simulink model "Generic_13"  (R2022b)
settings: Solver=VariableStepAuto  StartTime=0.0  StopTime=10.0  RelTol=1e-3
values from neighbouring files (symbols this model uses):
  A = cell2mat(A_cell)    [MPCController1.m]    (also in MPC_Fmincon.m)
  B = cell2mat(B_cell)    [MPCController1.m]    (also in MPC_Fmincon.m)
  brake_select = ones(length(speed), length(steering_angle))    [TwoDLook_uptable.m]
  curvature = 0.000:0.001:1    [TwoDLook_uptable.m]
  m = 1600    [MPCController1.m]    (also in MPCController2.m; MPC_Fmincon.m)
  speed = 0:0.1:100    [TwoDLook_uptable.m]
undefined symbols (not defined in the file or in its folder): Amplifier, DiscIntNeverNeededParam, K_d_yawrate, K_dsteering, k_speed, k_stanley, kd, ki, kp, path_curvature
libraries: CarMaker4SL x121, simulink x12, cstblocks x7, autolibshared x1, mpcadaslib x1
(part 3 of 5)

== system Generic_13/CreateBus VhclCtrl/Stanley  steering & speed//Brake controller/Road sensor set & path planning/Road sensor set & path planning/Dijkestra path planning/Signal_smoothing ==
  Signal_In : Inport
  Smoothing1 : Subsystem
  Smoothing2 : Subsystem
  Smoothing4 : Subsystem
  smoothed_width : Outport
  wires:
  Smoothing4/1(Signal_Out) -> smoothed_width/1  "smoothed_width"
  Smoothing2/1(Signal_Out) -> Smoothing4/1(Signal_In)  "steering_signal"
  Smoothing1/1(Signal_Out) -> Smoothing2/1(Signal_In)  "steering_signal"
  Signal_In/1 -> Smoothing1/1(Signal_In)

== system Generic_13/CreateBus VhclCtrl/Stanley  steering & speed//Brake controller/Road sensor set & path planning/Road sensor set & path planning/Dijkestra path planning/Smoothing3 ==
  Signal_In : Inport
  Add : Sum  Inputs=++++
  Delay : Delay  InitialCondition=0.1
  Delay1 : Delay  DelayLength=4  InitialCondition=0.1
  Delay2 : Delay  DelayLength=5  InitialCondition=0.1
  Gain : Gain  Gain=0.35
  Gain1 : Gain  Gain=0.25
  Gain2 : Gain  Gain=0.25
  Gain3 : Gain  Gain=0.15
  Signal_Out : Outport  VectorParamsAs1DForOutWhenUnconnected=off
  wires:
  Gain1/1 -> Add/2
  Signal_In/1 -> Gain/1
  Delay/1 -> Gain1/1
  Gain/1 -> Add/1
  Delay1/1 -> Gain2/1
  Add/1 -> Delay2/1, Delay1/1, Delay/1, Signal_Out/1
  Gain2/1 -> Add/3
  Delay2/1 -> Gain3/1
  Gain3/1 -> Add/4

== system Generic_13/CreateBus VhclCtrl/Stanley  steering & speed//Brake controller/Road sensor set & path planning/Road sensor set & path planning/Path_curvature/ Path_expanding ==
  X-path : Inport
  Y_path : Inport  Port=2
  Delay10 : Delay  DelayLength=6
  Delay11 : Delay  DelayLength=8
  Delay37 : Delay
  Delay38 : Delay  DelayLength=4
  Delay4 : Delay
  Delay5 : Delay  DelayLength=6
  Delay6 : Delay  DelayLength=8
  Delay9 : Delay  DelayLength=4
  Mux1 : Mux  Inputs=5
  Mux2 : Mux  Inputs=5
  Reshape1 : Reshape  OutputDimensionality=Customize  OutputDimensions=[1,5]
  Reshape2 : Reshape  OutputDimensionality=Customize  OutputDimensions=[1,5]
  x_path : Outport
  y_path : Outport  Port=2
  wires:
  X-path/1 -> Mux2/1, Delay38/1, Delay37/1, Delay5/1, Delay6/1
  Y_path/1 -> Mux1/1, Delay4/1, Delay9/1, Delay10/1, Delay11/1
  Delay5/1 -> Mux2/4
  Delay37/1 -> Mux2/2
  Delay6/1 -> Mux2/5
  Delay38/1 -> Mux2/3
  Mux1/1 -> Reshape1/1
  Reshape1/1 -> y_path/1
  Delay4/1 -> Mux1/2
  Delay9/1 -> Mux1/3
  Delay10/1 -> Mux1/4
  Delay11/1 -> Mux1/5
  Reshape2/1 -> x_path/1
  Mux2/1 -> Reshape2/1

== system Generic_13/CreateBus VhclCtrl/Stanley  steering & speed//Brake controller/Road sensor set & path planning/Road sensor set & path planning/Spline_path_planning/Signal_smoothing ==
  Signal_In : Inport
  Smoothing1 : Subsystem
  Smoothing2 : Subsystem
  Smoothing4 : Subsystem
  smoothed_width : Outport
  wires:
  Signal_In/1 -> Smoothing1/1(Signal_In)
  Smoothing1/1(Signal_Out) -> Smoothing2/1(Signal_In)  "steering_signal"
  Smoothing2/1(Signal_Out) -> Smoothing4/1(Signal_In)  "steering_signal"
  Smoothing4/1(Signal_Out) -> smoothed_width/1  "smoothed_width"

== system Generic_13/CreateBus VhclCtrl/Stanley  steering & speed//Brake controller/Road sensor set & path planning/Road sensor set & path planning/Spline_path_planning/Smoothing3 ==
  Signal_In : Inport
  Add : Sum  Inputs=++++
  Delay : Delay  InitialCondition=0.1
  Delay1 : Delay  DelayLength=4  InitialCondition=0.1
  Delay2 : Delay  DelayLength=5  InitialCondition=0.1
  Gain : Gain  Gain=0.35
  Gain1 : Gain  Gain=0.25
  Gain2 : Gain  Gain=0.25
  Gain3 : Gain  Gain=0.15
  Signal_Out : Outport  VectorParamsAs1DForOutWhenUnconnected=off
  wires:
  Gain3/1 -> Add/4
  Delay2/1 -> Gain3/1
  Gain2/1 -> Add/3
  Add/1 -> Signal_Out/1, Delay/1, Delay1/1, Delay2/1
  Delay1/1 -> Gain2/1
  Gain/1 -> Add/1
  Delay/1 -> Gain1/1
  Signal_In/1 -> Gain/1
  Gain1/1 -> Add/2

== system Generic_13/CreateBus VhclCtrl/Stanley  steering & speed//Brake controller/Road sensor set & path planning/Road sensor set & path planning/path_planning/Signal_smoothing ==
  Signal_In : Inport
  Smoothing1 : Subsystem
  Smoothing2 : Subsystem
  Smoothing4 : Subsystem
  smoothed_width : Outport
  wires:
  Smoothing4/1(Signal_Out) -> smoothed_width/1  "smoothed_width"
  Smoothing2/1(Signal_Out) -> Smoothing4/1(Signal_In)  "steering_signal"
  Smoothing1/1(Signal_Out) -> Smoothing2/1(Signal_In)  "steering_signal"
  Signal_In/1 -> Smoothing1/1(Signal_In)

== system Generic_13/CreateBus VhclCtrl/Stanley  steering & speed//Brake controller/Road sensor set & path planning/Road sensor set & path planning/path_planning/Smoothing3 ==
  Signal_In : Inport
  Add : Sum  Inputs=++++
  Delay : Delay  InitialCondition=0.1
  Delay1 : Delay  DelayLength=4  InitialCondition=0.1
  Delay2 : Delay  DelayLength=5  InitialCondition=0.1
  Gain : Gain  Gain=0.35
  Gain1 : Gain  Gain=0.25
  Gain2 : Gain  Gain=0.25
  Gain3 : Gain  Gain=0.15
  Signal_Out : Outport  VectorParamsAs1DForOutWhenUnconnected=off
  wires:
  Gain1/1 -> Add/2
  Signal_In/1 -> Gain/1
  Delay/1 -> Gain1/1
  Gain/1 -> Add/1
  Delay1/1 -> Gain2/1
  Add/1 -> Delay2/1, Delay1/1, Delay/1, Signal_Out/1
  Gain2/1 -> Add/3
  Delay2/1 -> Gain3/1
  Gain3/1 -> Add/4

== system Generic_13/CreateBus VhclCtrl/Stanley  steering & speed//Brake controller/Stanley_controller_vfin/Stanley_controller_vfin/Stanley_standfort controller/Crosstrack_steering ==
  speed : Inport
  Path.DevDist : Inport  Port=2
  Atan : Trigonometry  Operator=atan
  Divide : Product  Inputs=*/
  Gain : Gain  Gain=-1
  Product : Product
  Sum1 : Sum  Inputs=|++
  k_speed : Constant  Value=k_speed
  k_stanley : Constant  Value=k_stanley
  Cross_track_steering : Outport
  wires:
  Atan/1 -> Cross_track_steering/1
  Divide/1 -> Atan/1
  k_speed/1 -> Sum1/1
  speed/1 -> Sum1/2
  k_stanley/1 -> Product/2
  Sum1/1 -> Divide/2
  Product/1 -> Gain/1
  Gain/1 -> Divide/1
  Path.DevDist/1 -> Product/1

== system Generic_13/CreateBus VhclCtrl/Stanley  steering & speed//Brake controller/Stanley_controller_vfin/Stanley_controller_vfin/Stanley_standfort controller/Deviation_angle_calc ==
  Velocity : Inport
  Curvature : Inport  Port=2
  Car.YawRate : Inport  Port=3
  Amplifyer : Gain  Gain=Amplifier
  Amplifyer1 : Gain  Gain=10
  Amplifyer2 : Gain  Gain=16.56
  Constant : Constant  Value=2
  Discrete-Time Integrator : DiscreteIntegrator  SampleTime=-1  ICPrevOutput=DiscIntNeverNeededParam  ICPrevScaledInput=DiscIntNeverNeededParam
  Integrator : DiscreteIntegrator  SampleTime=-1  ICPrevOutput=DiscIntNeverNeededParam  ICPrevScaledInput=DiscIntNeverNeededParam
  Multiport Switch : MultiPortSwitch  Inputs=2  SaturateOnIntegerOverflow=off  InputSameDT=off
  Product : Product
  Read CM Dict : CarMaker4SL/Read CM Dict  xname=Sensor.Road.VehSensor_0.Path.DevAng  xsync=off  xstime=Continuous
  Scope : Scope  NumInputPorts=2
  Sum3 : Sum  Inputs=|+-
  Switch : Switch  Criteria=u2 > Threshold  SaturateOnIntegerOverflow=off  InputSameDT=off
  Dev_angle : Outport
  wires:
  Amplifyer1/1 -> Switch/3  "Dev_angle"
  Curvature/1 -> Product/1
  Car.YawRate/1 -> Discrete-Time Integrator/1
  Velocity/1 -> Product/2
  Product/1 -> Integrator/1
  Integrator/1 -> Sum3/1  "Dev_angle"
  Discrete-Time Integrator/1 -> Sum3/2
  Amplifyer2/1 -> Switch/1  "Dev_angle"
  Sum3/1 -> Amplifyer1/1, Switch/2, Amplifyer2/1  "heading_error"
  Switch/1 -> Scope/1, Multiport Switch/2  "Dev_angle"
  Amplifyer/1 -> Scope/2, Multiport Switch/3  "Dev_angle"
  Read CM Dict/1 -> Amplifyer/1
  Constant/1 -> Multiport Switch/1
  Multiport Switch/1 -> Dev_angle/1  "Dev_angle"

== system Generic_13/CreateBus VhclCtrl/Stanley  steering & speed//Brake controller/Stanley_controller_vfin/Stanley_controller_vfin/Stanley_standfort controller/Steady_state_yaw ==
  V : Inport
  Curvature : Inport  Port=2
  Car_Yaw_rate : Inport  Port=3
  Discrete-Time Integrator : DiscreteIntegrator  SampleTime=-1  ICPrevOutput=DiscIntNeverNeededParam  ICPrevScaledInput=DiscIntNeverNeededParam
  Steady_state_yaw : Subsystem
  Sum : Sum  Inputs=|-+
  Steady_state_yaw1 : Outport
  wires:
  V/1 -> Steady_state_yaw/1(V)
  Sum/1 -> Steady_state_yaw1/1  "Steady_state_yaw"
  Steady_state_yaw/1(Steady_state_yaw) -> Sum/1  "Steady_state_yaw"
  Discrete-Time Integrator/1 -> Sum/2
  Car_Yaw_rate/1 -> Discrete-Time Integrator/1
  Curvature/1 -> Steady_state_yaw/2(Curvature)

== system Generic_13/CreateBus VhclCtrl/Stanley  steering & speed//Brake controller/Stanley_controller_vfin/Stanley_controller_vfin/Stanley_standfort controller/Steering_correction_facotr ==
  Steering_i+1 : Inport
  Steering_i : Inport  Port=2
  K_dsteering : Constant  Value=K_dsteering
  Memory : Memory  LinearizeAsDelay=on
  Product2 : Product
  Sum2 : Sum  Inputs=|+-
  Factor_of_correction : Outport
  wires:
  K_dsteering/1 -> Product2/1
  Memory/1 -> Sum2/1
  Sum2/1 -> Product2/2
  Steering_i+1/1 -> Sum2/2
  Steering_i/1 -> Memory/1
  Product2/1 -> Factor_of_correction/1

== system Generic_13/CreateBus VhclCtrl/Stanley  steering & speed//Brake controller/Stanley_controller_vfin/Stanley_controller_vfin/Stanley_standfort controller/Yaw_rate_diff ==
  Velocity : Inport
  Curvature : Inport  Port=2
  Car_yaw_rate : Inport  Port=3
  K_d_yawrate : Constant  Value=K_d_yawrate
  Product : Product
  Product1 : Product
  Sum1 : Sum  Inputs=|+-
  Yaw_rate_factor : Outport
  wires:
  K_d_yawrate/1 -> Product1/1
  Car_yaw_rate/1 -> Sum1/2
  Velocity/1 -> Product/1
  Curvature/1 -> Product/2
  Sum1/1 -> Product1/2
  Product/1 -> Sum1/1
  Product1/1 -> Yaw_rate_factor/1

== system Generic_13/CreateBus VhclCtrl/Stanley  steering & speed//Brake controller/Road sensor set & path planning/Road sensor set & path planning/A* star path planning/Signal_smoothing/Smoothing1 ==
  Signal_In : Inport
  Add : Sum  Inputs=++++
  Delay : Delay  InitialCondition=0.1
  Delay1 : Delay  DelayLength=4  InitialCondition=0.1
  Delay2 : Delay  DelayLength=5  InitialCondition=0.1
  Gain : Gain  Gain=0.35
  Gain1 : Gain  Gain=0.25
  Gain2 : Gain  Gain=0.25
  Gain3 : Gain  Gain=0.15
  Signal_Out : Outport  VectorParamsAs1DForOutWhenUnconnected=off
  wires:
  Gain1/1 -> Add/2
  Signal_In/1 -> Gain/1
  Delay/1 -> Gain1/1
  Gain/1 -> Add/1
  Delay1/1 -> Gain2/1
  Add/1 -> Delay2/1, Delay1/1, Delay/1, Signal_Out/1
  Gain2/1 -> Add/3
  Delay2/1 -> Gain3/1
  Gain3/1 -> Add/4

== system Generic_13/CreateBus VhclCtrl/Stanley  steering & speed//Brake controller/Road sensor set & path planning/Road sensor set & path planning/A* star path planning/Signal_smoothing/Smoothing2 ==
  Signal_In : Inport
  Add : Sum  Inputs=++++
  Delay : Delay  InitialCondition=0.1
  Delay1 : Delay  DelayLength=4  InitialCondition=0.1
  Delay2 : Delay  DelayLength=5  InitialCondition=0.1
  Gain : Gain  Gain=0.35
  Gain1 : Gain  Gain=0.25
  Gain2 : Gain  Gain=0.25
  Gain3 : Gain  Gain=0.15
  Signal_Out : Outport  VectorParamsAs1DForOutWhenUnconnected=off
  wires:
  Gain3/1 -> Add/4
  Delay2/1 -> Gain3/1
  Gain2/1 -> Add/3
  Add/1 -> Signal_Out/1, Delay/1, Delay1/1, Delay2/1
  Delay1/1 -> Gain2/1
  Gain/1 -> Add/1
  Delay/1 -> Gain1/1
  Signal_In/1 -> Gain/1
  Gain1/1 -> Add/2

== system Generic_13/CreateBus VhclCtrl/Stanley  steering & speed//Brake controller/Road sensor set & path planning/Road sensor set & path planning/A* star path planning/Signal_smoothing/Smoothing4 ==
  Signal_In : Inport
  Add : Sum  Inputs=++++
  Delay : Delay  InitialCondition=0.1
  Delay1 : Delay  DelayLength=4  InitialCondition=0.1
  Delay2 : Delay  DelayLength=5  InitialCondition=0.1
  Gain : Gain  Gain=0.35
  Gain1 : Gain  Gain=0.25
  Gain2 : Gain  Gain=0.25
  Gain3 : Gain  Gain=0.15
  Signal_Out : Outport  VectorParamsAs1DForOutWhenUnconnected=off
  wires:
  Gain1/1 -> Add/2
  Signal_In/1 -> Gain/1
  Delay/1 -> Gain1/1
  Gain/1 -> Add/1
  Delay1/1 -> Gain2/1
  Add/1 -> Delay2/1, Delay1/1, Delay/1, Signal_Out/1
  Gain2/1 -> Add/3
  Delay2/1 -> Gain3/1
  Gain3/1 -> Add/4

== system Generic_13/CreateBus VhclCtrl/Stanley  steering & speed//Brake controller/Road sensor set & path planning/Road sensor set & path planning/Be'zeir path planning/Signal_smoothing/Smoothing1 ==
  Signal_In : Inport
  Add : Sum  Inputs=++++
  Delay : Delay  InitialCondition=0.1
  Delay1 : Delay  DelayLength=4  InitialCondition=0.1
  Delay2 : Delay  DelayLength=5  InitialCondition=0.1
  Gain : Gain  Gain=0.35
  Gain1 : Gain  Gain=0.25
  Gain2 : Gain  Gain=0.25
  Gain3 : Gain  Gain=0.15
  Signal_Out : Outport  VectorParamsAs1DForOutWhenUnconnected=off
  wires:
  Gain3/1 -> Add/4
  Delay2/1 -> Gain3/1
  Gain2/1 -> Add/3
  Add/1 -> Signal_Out/1, Delay/1, Delay1/1, Delay2/1
  Delay1/1 -> Gain2/1
  Gain/1 -> Add/1
  Delay/1 -> Gain1/1
  Signal_In/1 -> Gain/1
  Gain1/1 -> Add/2

== system Generic_13/CreateBus VhclCtrl/Stanley  steering & speed//Brake controller/Road sensor set & path planning/Road sensor set & path planning/Be'zeir path planning/Signal_smoothing/Smoothing2 ==
  Signal_In : Inport
  Add : Sum  Inputs=++++
  Delay : Delay  InitialCondition=0.1
  Delay1 : Delay  DelayLength=4  InitialCondition=0.1
  Delay2 : Delay  DelayLength=5  InitialCondition=0.1
  Gain : Gain  Gain=0.35
  Gain1 : Gain  Gain=0.25
  Gain2 : Gain  Gain=0.25
  Gain3 : Gain  Gain=0.15
  Signal_Out : Outport  VectorParamsAs1DForOutWhenUnconnected=off
  wires:
  Gain1/1 -> Add/2
  Signal_In/1 -> Gain/1
  Delay/1 -> Gain1/1
  Gain/1 -> Add/1
  Delay1/1 -> Gain2/1
  Add/1 -> Delay2/1, Delay1/1, Delay/1, Signal_Out/1
  Gain2/1 -> Add/3
  Delay2/1 -> Gain3/1
  Gain3/1 -> Add/4

== system Generic_13/CreateBus VhclCtrl/Stanley  steering & speed//Brake controller/Road sensor set & path planning/Road sensor set & path planning/Be'zeir path planning/Signal_smoothing/Smoothing4 ==
  Signal_In : Inport
  Add : Sum  Inputs=++++
  Delay : Delay  InitialCondition=0.1
  Delay1 : Delay  DelayLength=4  InitialCondition=0.1
  Delay2 : Delay  DelayLength=5  InitialCondition=0.1
  Gain : Gain  Gain=0.35
  Gain1 : Gain  Gain=0.25
  Gain2 : Gain  Gain=0.25
  Gain3 : Gain  Gain=0.15
  Signal_Out : Outport  VectorParamsAs1DForOutWhenUnconnected=off
  wires:
  Gain3/1 -> Add/4
  Delay2/1 -> Gain3/1
  Gain2/1 -> Add/3
  Add/1 -> Signal_Out/1, Delay/1, Delay1/1, Delay2/1
  Delay1/1 -> Gain2/1
  Gain/1 -> Add/1
  Delay/1 -> Gain1/1
  Signal_In/1 -> Gain/1
  Gain1/1 -> Add/2

== system Generic_13/CreateBus VhclCtrl/Stanley  steering & speed//Brake controller/Road sensor set & path planning/Road sensor set & path planning/Dijkestra path planning/Signal_smoothing/Smoothing1 ==
  Signal_In : Inport
  Add : Sum  Inputs=++++
  Delay : Delay  InitialCondition=0.1
  Delay1 : Delay  DelayLength=4  InitialCondition=0.1
  Delay2 : Delay  DelayLength=5  InitialCondition=0.1
  Gain : Gain  Gain=0.35
  Gain1 : Gain  Gain=0.25
  Gain2 : Gain  Gain=0.25
  Gain3 : Gain  Gain=0.15
  Signal_Out : Outport  VectorParamsAs1DForOutWhenUnconnected=off
  wires:
  Gain3/1 -> Add/4
  Delay2/1 -> Gain3/1
  Gain2/1 -> Add/3
  Add/1 -> Signal_Out/1, Delay/1, Delay1/1, Delay2/1
  Delay1/1 -> Gain2/1
  Gain/1 -> Add/1
  Delay/1 -> Gain1/1
  Signal_In/1 -> Gain/1
  Gain1/1 -> Add/2

== system Generic_13/CreateBus VhclCtrl/Stanley  steering & speed//Brake controller/Road sensor set & path planning/Road sensor set & path planning/Dijkestra path planning/Signal_smoothing/Smoothing2 ==
  Signal_In : Inport
  Add : Sum  Inputs=++++
  Delay : Delay  InitialCondition=0.1
  Delay1 : Delay  DelayLength=4  InitialCondition=0.1
  Delay2 : Delay  DelayLength=5  InitialCondition=0.1
  Gain : Gain  Gain=0.35
  Gain1 : Gain  Gain=0.25
  Gain2 : Gain  Gain=0.25
  Gain3 : Gain  Gain=0.15
  Signal_Out : Outport  VectorParamsAs1DForOutWhenUnconnected=off
  wires:
  Gain1/1 -> Add/2
  Signal_In/1 -> Gain/1
  Delay/1 -> Gain1/1
  Gain/1 -> Add/1
  Delay1/1 -> Gain2/1
  Add/1 -> Delay2/1, Delay1/1, Delay/1, Signal_Out/1
  Gain2/1 -> Add/3
  Delay2/1 -> Gain3/1
  Gain3/1 -> Add/4

== system Generic_13/CreateBus VhclCtrl/Stanley  steering & speed//Brake controller/Road sensor set & path planning/Road sensor set & path planning/Dijkestra path planning/Signal_smoothing/Smoothing4 ==
  Signal_In : Inport
  Add : Sum  Inputs=++++
  Delay : Delay  InitialCondition=0.1
  Delay1 : Delay  DelayLength=4  InitialCondition=0.1
  Delay2 : Delay  DelayLength=5  InitialCondition=0.1
  Gain : Gain  Gain=0.35
  Gain1 : Gain  Gain=0.25
  Gain2 : Gain  Gain=0.25
  Gain3 : Gain  Gain=0.15
  Signal_Out : Outport  VectorParamsAs1DForOutWhenUnconnected=off
  wires:
  Gain3/1 -> Add/4
  Delay2/1 -> Gain3/1
  Gain2/1 -> Add/3
  Add/1 -> Signal_Out/1, Delay/1, Delay1/1, Delay2/1
  Delay1/1 -> Gain2/1
  Gain/1 -> Add/1
  Delay/1 -> Gain1/1
  Signal_In/1 -> Gain/1
  Gain1/1 -> Add/2

== system Generic_13/CreateBus VhclCtrl/Stanley  steering & speed//Brake controller/Road sensor set & path planning/Road sensor set & path planning/Spline_path_planning/Signal_smoothing/Smoothing1 ==
  Signal_In : Inport
  Add : Sum  Inputs=++++
  Delay : Delay  InitialCondition=0.1
  Delay1 : Delay  DelayLength=4  InitialCondition=0.1
  Delay2 : Delay  DelayLength=5  InitialCondition=0.1
  Gain : Gain  Gain=0.35
  Gain1 : Gain  Gain=0.25
  Gain2 : Gain  Gain=0.25
  Gain3 : Gain  Gain=0.15
  Signal_Out : Outport  VectorParamsAs1DForOutWhenUnconnected=off
  wires:
  Gain1/1 -> Add/2
  Signal_In/1 -> Gain/1
  Delay/1 -> Gain1/1
  Gain/1 -> Add/1
  Delay1/1 -> Gain2/1
  Add/1 -> Delay2/1, Delay1/1, Delay/1, Signal_Out/1
  Gain2/1 -> Add/3
  Delay2/1 -> Gain3/1
  Gain3/1 -> Add/4

== system Generic_13/CreateBus VhclCtrl/Stanley  steering & speed//Brake controller/Road sensor set & path planning/Road sensor set & path planning/Spline_path_planning/Signal_smoothing/Smoothing2 ==
  Signal_In : Inport
  Add : Sum  Inputs=++++
  Delay : Delay  InitialCondition=0.1
  Delay1 : Delay  DelayLength=4  InitialCondition=0.1
  Delay2 : Delay  DelayLength=5  InitialCondition=0.1
  Gain : Gain  Gain=0.35
  Gain1 : Gain  Gain=0.25
  Gain2 : Gain  Gain=0.25
  Gain3 : Gain  Gain=0.15
  Signal_Out : Outport  VectorParamsAs1DForOutWhenUnconnected=off
  wires:
  Gain3/1 -> Add/4
  Delay2/1 -> Gain3/1
  Gain2/1 -> Add/3
  Add/1 -> Signal_Out/1, Delay/1, Delay1/1, Delay2/1
  Delay1/1 -> Gain2/1
  Gain/1 -> Add/1
  Delay/1 -> Gain1/1
  Signal_In/1 -> Gain/1
  Gain1/1 -> Add/2

== system Generic_13/CreateBus VhclCtrl/Stanley  steering & speed//Brake controller/Road sensor set & path planning/Road sensor set & path planning/Spline_path_planning/Signal_smoothing/Smoothing4 ==
  Signal_In : Inport
  Add : Sum  Inputs=++++
  Delay : Delay  InitialCondition=0.1
  Delay1 : Delay  DelayLength=4  InitialCondition=0.1
  Delay2 : Delay  DelayLength=5  InitialCondition=0.1
  Gain : Gain  Gain=0.35
  Gain1 : Gain  Gain=0.25
  Gain2 : Gain  Gain=0.25
  Gain3 : Gain  Gain=0.15
  Signal_Out : Outport  VectorParamsAs1DForOutWhenUnconnected=off
  wires:
  Gain1/1 -> Add/2
  Signal_In/1 -> Gain/1
  Delay/1 -> Gain1/1
  Gain/1 -> Add/1
  Delay1/1 -> Gain2/1
  Add/1 -> Delay2/1, Delay1/1, Delay/1, Signal_Out/1
  Gain2/1 -> Add/3
  Delay2/1 -> Gain3/1
  Gain3/1 -> Add/4

== system Generic_13/CreateBus VhclCtrl/Stanley  steering & speed//Brake controller/Road sensor set & path planning/Road sensor set & path planning/path_planning/Signal_smoothing/Smoothing1 ==
  Signal_In : Inport
  Add : Sum  Inputs=++++
  Delay : Delay  InitialCondition=0.1
  Delay1 : Delay  DelayLength=4  InitialCondition=0.1
  Delay2 : Delay  DelayLength=5  InitialCondition=0.1
  Gain : Gain  Gain=0.35
  Gain1 : Gain  Gain=0.25
  Gain2 : Gain  Gain=0.25
  Gain3 : Gain  Gain=0.15
  Signal_Out : Outport  VectorParamsAs1DForOutWhenUnconnected=off
  wires:
  Gain3/1 -> Add/4
  Delay2/1 -> Gain3/1
  Gain2/1 -> Add/3
  Add/1 -> Signal_Out/1, Delay/1, Delay1/1, Delay2/1
  Delay1/1 -> Gain2/1
  Gain/1 -> Add/1
  Delay/1 -> Gain1/1
  Signal_In/1 -> Gain/1
  Gain1/1 -> Add/2

== system Generic_13/CreateBus VhclCtrl/Stanley  steering & speed//Brake controller/Road sensor set & path planning/Road sensor set & path planning/path_planning/Signal_smoothing/Smoothing2 ==
  Signal_In : Inport
  Add : Sum  Inputs=++++
  Delay : Delay  InitialCondition=0.1
  Delay1 : Delay  DelayLength=4  InitialCondition=0.1
  Delay2 : Delay  DelayLength=5  InitialCondition=0.1
  Gain : Gain  Gain=0.35
  Gain1 : Gain  Gain=0.25
  Gain2 : Gain  Gain=0.25
  Gain3 : Gain  Gain=0.15
  Signal_Out : Outport  VectorParamsAs1DForOutWhenUnconnected=off
  wires:
  Gain1/1 -> Add/2
  Signal_In/1 -> Gain/1
  Delay/1 -> Gain1/1
  Gain/1 -> Add/1
  Delay1/1 -> Gain2/1
  Add/1 -> Delay2/1, Delay1/1, Delay/1, Signal_Out/1
  Gain2/1 -> Add/3
  Delay2/1 -> Gain3/1
  Gain3/1 -> Add/4

== system Generic_13/CreateBus VhclCtrl/Stanley  steering & speed//Brake controller/Road sensor set & path planning/Road sensor set & path planning/path_planning/Signal_smoothing/Smoothing4 ==
  Signal_In : Inport
  Add : Sum  Inputs=++++
  Delay : Delay  InitialCondition=0.1
  Delay1 : Delay  DelayLength=4  InitialCondition=0.1
  Delay2 : Delay  DelayLength=5  InitialCondition=0.1
  Gain : Gain  Gain=0.35
  Gain1 : Gain  Gain=0.25
  Gain2 : Gain  Gain=0.25
  Gain3 : Gain  Gain=0.15
  Signal_Out : Outport  VectorParamsAs1DForOutWhenUnconnected=off
  wires:
  Gain3/1 -> Add/4
  Delay2/1 -> Gain3/1
  Gain2/1 -> Add/3
  Add/1 -> Signal_Out/1, Delay/1, Delay1/1, Delay2/1
  Delay1/1 -> Gain2/1
  Gain/1 -> Add/1
  Delay/1 -> Gain1/1
  Signal_In/1 -> Gain/1
  Gain1/1 -> Add/2

== system Generic_13/CreateBus VhclCtrl/Stanley  steering & speed//Brake controller/Stanley_controller_vfin/Stanley_controller_vfin/Stanley_standfort controller/Steady_state_yaw/Steady_state_yaw ==
  V : Inport
  Curvature : Inport  Port=2
  Constant : Constant  Value=1600.004
  Constant1 : Constant  Value=70551.0
  Constant3 : Constant  Value=1.488
  Constant4 : Constant  Value=1.487
  Constant5 : Constant
  Divide : Product  Inputs=*/
  Divide1 : Product  Inputs=*/
  Gain : Gain  Gain=180/pi()
  Product : Product  Inputs=3
  Product1 : Product
  Square : Math  Operator=square
  Sum : Sum  Inputs=|++
  Steady_state_yaw : Outport
  wires:
  Square/1 -> Product/1
  Constant4/1 -> Divide/1
  Constant5/1 -> Sum/1
  Constant3/1 -> Divide/2
  V/1 -> Square/1
  Divide/1 -> Sum/2
  Sum/1 -> Product1/2
  Constant/1 -> Product/2
  Curvature/1 -> Product/3
  Constant1/1 -> Gain/1
  Product/1 -> Divide1/1
  Product1/1 -> Divide1/2
  Divide1/1 -> Steady_state_yaw/1
  Gain/1 -> Product1/1

== matlab function Generic_13/CreateBus VhclCtrl/MPC_steering_controllers/MATLAB Function1 ==
  data: dev input; steering output; B input
function steering = advanced_speed_control_mpc(dev,B)
    % Model Predictive Controller (MPC) for speed contol
    % Define MPC parameters
    Ts = 0.1;  % Sampling time
    N = 10;    % Prediction horizon
    Q = 1;     % State weight
    R = 1;     % Input weight
    S = 0.1;   % Terminal state weight (integral term)
    
    % State-space model (simplified for illustration)
    %A = 0.8;
    %B = Ts;
    
    % Define cost and constraints for fmincon
    costFunction = @(u) (dev + B * u)' * Q * (dev + B * u) + u' * R * u + S * sum(u);
    Aeq = [];
    Beq = [];
    Aineq = [];
    Bineq = [];
    lb = -3.14; % Lower bound on throttle
    ub = 3.14;  % Upper bound on throttle
    
    % Steady-state error constraint
    Aineq = [Aineq; B];
    Bineq = [Bineq; -dev];
    
    % Initial guess
    u0 = 0;
    
    % Solve optimization problem
    options = optimoptions('fmincon', 'Display', 'off', 'Algorithm', 'sqp');
    u_opt = fmincon(costFunction, u0, Aineq, Bineq, Aeq, Beq, lb, ub, [], options);
    
    % Extract control input (throttle) from the optimization result
    steering = u_opt;
end

== matlab function Generic_13/CreateBus VhclCtrl/Stanley  steering & speed//Brake controller/Stanley_controller_with_thottle_and_brake_commands/Stanley steering + PID speed controller/Speed_controller/calculate_path_curvature ==
  data: path input; path_curvature output size=[1 20]; min_safe_speed output size=[1 20]; velocity_y input; velocity_x input; steering_angel input
function [path_curvature, min_safe_speed] = calculate_path_curvature(path,velocity_y,velocity_x,steering_angel)
    v_x = velocity_x* ones(1,20);
    v_y = velocity_y*ones(1,20);
    x = path(1,:)+v_x;
    y = path(2,:)+v_y;
    % First and second derivatives
    dx = gradient(x);
    dy = gradient(y);
    
    ddx = gradient(dx);
    ddy = gradient(dy);
    
    % Path curvature
    path_curvature = (dx .* ddy - dy .* ddx) ./ (dx.^2 + dy.^2).^(3/2);
    R = sqrt(1.61^2 +(1.61+1.28)^2*cot(steering_angel)^2)/12;
    % Minimum safe speed
    g = 9.81; % gravitational acceleration
    if max(path_curvature)>0.001 || max(path_curvature)<-0.001

        min_safe_speed = sqrt(g ./ abs(path_curvature));
    else
        min_safe_speed = sqrt(g .* abs(path_curvature));
end

== matlab function Generic_13/CreateBus VhclCtrl/Stanley  steering & speed//Brake controller/Stanley_controller_with_thottle_and_brake_commands/Stanley steering + PID speed controller/Stanely_controller ==
  data: dev_angle input; dev input; x1 input; x2 input; y1 input; y2 input; speed_act input; e output; cross_track_steering output; steering output
function [e, cross_track_steering, steering]  = conversion(dev_angle,dev, x1,x2,y1,y2,speed_act)


e = zeros(1);
cross_track_steering = zeros(1);


k_exp = 1.36;
k_def = 6;
k = k_def + abs(speed_act)^k_exp;

% Perform linear regression to find a, b, and c
% X = [path(1, :); path(2, :); ones(1, 20)]';  % Create a matrix for linear regression
% coefficients = X \ -1 * ones(20, 1);
% 
% % Extract the coefficients a, b, and c
% a = coefficients(1);
% b = coefficients(2);
% c = coefficients(3);
if (x2 ==0 && x1 ==0)|| x2==x1
a = 0;
b = 1;
c = y2+a*x2;
else
a = -(y2 - y1)/(x2-x1);
b = 1;
c = y2+a*x2;
end

if speed_act ~=0
    %e =abs(a*x_car+b*y_car+c)\sqrt(a^2+b^2); %abs(Dev_dis);
    e =-1*dev;% deviation distance
    cross_track_steering = atan(e*k / (1+speed_act));
    %heading_err = atan(-a/b)-yaw;
    heading_err = dev_angle; % heading error OR deviation angle
    steering = heading_err + cross_track_steering;

else
    steering = 0;
end
end

== matlab function Generic_13/CreateBus VhclCtrl/MPC_steering_controllers/MATLAB Function2 ==
  data: x_car input; target_heading output; y_car input; x_path input; y_path input; yaw_angle input; current_heading output
function [target_heading, current_heading] = calculate_headings(x_car, y_car, x_path, y_path, yaw_angle)
    % Calculate headings based on car and path positions and yaw angle
    function angle = normalize_angle(angle)
    % Normalize an angle to be in the range [-pi, pi]
    while angle > pi
        angle = angle - 2*pi;
    end

    while angle < -pi
        angle = angle + 2*pi;
    end
end
    % Calculate angle from car to path (target_heading)
    target_heading = atan2(y_path - y_car, x_path - x_car);
    
    % Adjust yaw angle to be in the range [-pi, pi]
    yaw_angle = normalize_angle(yaw_angle);
    
    % Current heading is the yaw angle of the vehicle
    current_heading = yaw_angle;
end

== matlab function Generic_13/CreateBus VhclCtrl/Stanley  steering & speed//Brake controller/Stanley_controller_with_thottle_and_brake_commands/Stanley steering + PID speed controller/Subsystem1/MATLAB Function ==
  data: u input; curv output; min_safe_speed input; speed output
function [curv, speed] = fcn(u, min_safe_speed)

curv = abs(max(u));
speed = max(min_safe_speed);

== matlab function Generic_13/CreateBus VhclCtrl/MPC_steering_controllers/MATLAB Function3 ==
  data: target_heading input; delta output; current_heading input; dt input; vx input; vy input
function delta = adaptive_steering_mpc(target_heading, current_heading, dt,vx,vy)
    % Adaptive Model Predictive Controller (Adaptive MPC) for steering control
    function dx = calculate_dynamics(u, m, l, Iz, dt, vx, vy)
    % Calculate the dynamics of the system (Bicycle Model)

    % Unpack state variables
    vy1 = vy - l * u;  % Correct lateral velocity for the tire slip angle

    % Bicycle model equations
    a = (2 * (u - vy1)) / (m * vx);
    b = (2 * l * (u - vy1)) / Iz;

    % State dynamics
    dx1 = a * dt;
    dx2 = b * dt;

    % Update state variables
    dx = [dx1; dx2];
end
    % Define Q and R matrices
    Q = eye(2);  % Weighting matrix for state
    R = eye(1);  % Weighting matrix for control input

    % Define system parameters (replace these with your actual vehicle parameters)
    m = 1600;           % Vehicle mass [kg]
    l = 2.975;          % Wheelbase [m]
    Iz = 2986.624;      % Vehicle inertia [kg*m^2]
    
    % Adaptive parameters
    alpha = 0.1;  % Adaptation rate
    theta = [0.1; 0.1];  % Initial guess of parameters
    
    % State vector (simplified, assuming current_heading is the heading error)
    x = [current_heading; 0];
    
    % Define cost and constraints for fmincon
    costFunction = @(u) (x + calculate_dynamics(u, m, l, Iz, dt,vx,vy))' * Q * (x + calculate_dynamics(u, m, l, Iz, dt,vx,vy)) + u' * R * u;
    Aeq = [];
    Beq = [];
    Aineq = [];
    Bineq = [];
    lb = -1.6;  % Lower bound on steering input
    ub = 1.6;   % Upper bound on steering input
    
    % Initial guess
    u0 = 0.1;
    
    % Solve optimization problem to get optimal steering input
    options = optimoptions('fmincon', 'Display', 'off', 'Algorithm', 'sqp');
    u_opt = fmincon(costFunction, u0, Aineq, Bineq, Aeq, Beq, lb, ub, [], options);
    
    % Update adaptive parameters online (using a simple gradient descent)
    x_next = x + calculate_dynamics(u_opt, m, l, Iz, dt,vx,vy);
    theta = theta - alpha * (x_next - (x + calculate_dynamics(u_opt, m, l, Iz, dt,vx,vy))) * x';
    
    % Extract control input (steering angle) from the optimization result
    delta = u_opt;
end

== matlab function Generic_13/CreateBus VhclCtrl/MPC_steering_controllers/MATLAB Function4 ==
  data: target_heading input; delta output; current_heading input; dt input
function delta = mpc_steering_control(target_heading, current_heading, dt)
    % Model Predictive Controller (MPC) for steering control
    
    % Parameters
    Ts = 0.1;  % Sampling time
    N = 10;    % Prediction horizon
    
    % System dynamics (simplified for illustration)
    A = eye(2);  % State matrix (identity matrix for simplicity)
    B = [0; 1];  % Input matrix (represents steering input)
    
    % State vector (simplified, assuming current_heading is the heading error)
    x = [current_heading; 0];
    
    % Define cost and constraints for fmincon
    costFunction = @(u) (x + A * x + B * u)' * (x + A * x + B * u);
    Aeq = [];
    Beq = [];
    Aineq = [];
    Bineq = [];
    lb = -1.5;  % Lower bound on steering input
    ub = 1.5;   % Upper bound on steering input
    
    % Initial guess
    u0 = 0;
    
    % Solve optimization problem to get optimal steering input
    options = optimoptions('fmincon', 'Display', 'off', 'Algorithm', 'sqp');
    u_opt = fmincon(costFunction, u0, Aineq, Bineq, Aeq, Beq, lb, ub, [], options);
    
    % Extract control input (steering angle) from the optimization result
    delta = u_opt;
end

== matlab function Generic_13/CreateBus VhclCtrl/Stanley  steering & speed//Brake controller/Stanley controller with path_planning/Stanley controller with path_planning/Path_Calculation_V02 ==
  data: x_car input; closest_point output; y_car input; path_x input; instantaneous_path output; y_path input
function [closest_point, instantaneous_path] = calculate_path(x_car, y_car, path_x, y_path)
% x_car: x position of the car
% y_car: y position of the car
% path: [2x400] matrix representing the path
path = [path_x;y_path];
%Smoothing the Path
x = path(1,:);
y = path(2,:);
% Define the number of points you want to add for interpolation
num_extra_points = 10000; % Adjust this value as per your requirements
% Compute the total number of points after interpolation
total_points = numel(x) + num_extra_points;
existing_indices = 1:numel(x);
% Create an array of indices for the interpolated points
interpolated_indices = linspace(1, numel(x), total_points);
% Perform spline interpolation on both x and y coordinates
x_interpolated = spline(existing_indices, x, interpolated_indices);
y_interpolated = spline(existing_indices, y, interpolated_indices);

smoothed_path =vertcat(x_interpolated, y_interpolated);
% smoothed_path = smoothed_path_t';


% Calculate the distance between the car and each point on the path
distances = sqrt((smoothed_path(1,:) - x_car).^2 + (smoothed_path(2,:) - y_car).^2);

% Find the index of the closest point on the path
[~, closest_index] = min(distances);

% Get the closest point on the path
closest_point = smoothed_path(:, closest_index);

% Calculate the distance from the closest point to the beginning of the path
distance_to_start = sqrt(sum((smoothed_path(:,closest_index) - smoothed_path(:,1)).^2));

% Calculate the distance from the closest point to the end of the path
distance_to_end = sqrt(sum((smoothed_path(:,closest_index) - smoothed_path(:,end)).^2));

% Determine the number of points to include in the instantaneous path
num_points = min(size(smoothed_path, 2), 20);

% Initialize the instantaneous_path variable using coder.nullcopy
instantaneous_path = coder.nullcopy(zeros(2, num_points));

if distance_to_start < distance_to_end
    % If the closest point is closer to the beginning of the path than the
    % end, include the points starting from the closest point towards the
    % end of the path
    start_index = closest_index;
    end_index = min(size(smoothed_path, 2), closest_index+num_points-1);
else
    % If the closest point is closer to the end of the path than the
    % beginning, include the points starting from the closest point towards
    % the beginning of the path
    start_index = max(1, closest_index-num_points+1);
    end_index = closest_index;
end

%own 
start_index = closest_index;
if start_index > 11139
    end_index = 11159;
    if start_index > 11149
        start_index = 0;
        end_index=20;
    end
else
    end_index = min(size(smoothed_path, 2), closest_index+num_points-1);
end
%own

temp_path = smoothed_path(:, start_index:end_index);
instantaneous_path(:, num_points-size(temp_path, 2)+1:num_points) = temp_path;

end

== matlab function Generic_13/CreateBus VhclCtrl/Stanley  steering & speed//Brake controller/Stanley controller with path_planning/Stanley controller with path_planning/MATLAB Function1 ==
  data: Pos_X input; Path_Out output; Pos_Y input; Yaw_Angle input; Path_In input
function Path_Out = Abs2RelNew(Pos_X, Pos_Y, Yaw_Angle, Path_In)
%Rotation matrix from absolute to relativ coordination system
R = [cos(Yaw_Angle) sin(Yaw_Angle); -sin(Yaw_Angle) cos(Yaw_Angle)];

Path_X=Path_In(1,:)-Pos_X;      % Shift the points in to the car position
Path_Y=Path_In(2,:)-Pos_Y;      % Shift the points in to the car position
Path=[Path_X;Path_Y];           % Car Point
Path_Out = R*Path;              % Rotate the shifted Points

== matlab function Generic_13/CreateBus VhclCtrl/Obstacle_data_gathering/MATLAB Function6 ==
  data: path_dev input; error output; y_dev input; y_error3 input; y_error_2 input; y_error input; distance input; x_distance_obj input
function error= fcn(path_dev, y_dev, y_error3, y_error_2, y_error, distance, x_distance_obj)
if distance <15 && distance >1
    %if y_error >0 || y_error_2 >0 || y_error3 >0
    %error =-(path_dev+y_dev/2);
    %else
        error =path_dev-y_dev/2;
elseif distance <1 && distance >-4
    error =path_dev/4-y_dev/2;
elseif (distance <-5 && distance >-8) && x_distance_obj >0
    error = -path_dev/4;
elseif distance <-6 && distance >-11.5
    error = -path_dev + path_dev/1.69; % path_dev - something_ (positve->0 when the we are not near the object
else
    error = path_dev;
end
end

== matlab function Generic_13/CreateBus VhclCtrl/Obstacle_data_gathering/MATLAB Function8 ==
  data: y_added output; y_dev input; data input; distance input
function y_added= fcn( y_dev, data, distance)
if distance <12 && distance >-4
   y_added = data+y_dev;
else
    y_added = 0;
end
end

== matlab function Generic_13/CreateBus VhclCtrl/MATLAB Function1 ==
  data: e input; steering output; Cf input; Cr input; v input
function steering = fcn(e,Cf,Cr,v)
%lf = 1.488
%lr = 1.487;
%Cf = 
%Cr =
%m =
% v = 
steering = ((lf+lr)- (lf*Cf-lr*Cr)*m*vx^2)*e...
    /(d_pre*(d_pre+2*L));

== matlab function Generic_13/CreateBus VhclCtrl/path_planner_MATLAB/MATLAB Function1 ==
  data: u input; path_x output; path_y output; path_yaw output
function [path_x,path_y,path_yaw] = fcn(u)
path_x = u(1,:);
path_y = u(2,:);
path_yaw = u(3,:);
end

== matlab function Generic_13/CreateBus VhclCtrl/path_planner_MATLAB/MATLAB Function ==
  data: path input; e output; yaw input; speed_act input; err_fr_axle output; cross_track_steering output; heading_err output; steering output
function [e, err_fr_axle, cross_track_steering, heading_err, steering]  = conversion(path,yaw,speed_act)
%path = [path_x;path_y];
function distance = calc_distance(pt,v1,v2)
    vect = v1 - v2;
    p_to_vect = pt - v2;
    crossVP = cross(vect,p_to_vect);
    distance = norm(crossVP) / norm(vect) * crossVP(3)/abs(crossVP(3));
end

e = zeros(1);
cross_track_steering = zeros(1);
heading_err = zeros(1);
steering=zeros(1);
err_fr_axle = zeros(1);

k_exp = 1.36;
k_def = 6;
k = k_def + abs(speed_act)^k_exp;
k_ref = 3.1;

% path_index = fix(k_path * speed_act);
% if path_index > 13
%     path_index = 13;
% end
% 
% P_prev = path(:,6 + path_index);
% P_next = path(:,7 + path_index);

fr_axle = [-1.488 0 0];
distances = sqrt((path(1,:) - 1.488).^2 + (path(2,:) - 0).^2);
% Find the index of the closest point on the path
[~,err_fr_axle_ind] = min(distances);
if err_fr_axle_ind == 1
    err_fr_axle_ind = 2;
end
err_fr_axle = calc_distance(fr_axle,[path(1,err_fr_axle_ind - 1) path(2,err_fr_axle_ind - 1) 0],[path(1,err_fr_axle_ind) path(2,err_fr_axle_ind) 0]);

B = [-1.488 + k_ref * (speed_act / 27) 0 0];
distances_err = sqrt((path(1,:) - B(1)).^2 + (path(2,:) - 0).^2);
[~,err_ind] = min(distances_err);
if err_ind < 2
    err_ind = 2;
end
error = calc_distance(B,[path(1,err_ind - 1) path(2,err_ind - 1) 0],[path(1,err_ind) path(2,err_ind) 0]);


P_prev = path(:, err_ind-1);
P_next = path(:, err_ind);

x1 = P_prev(1,1);
y1 = P_prev(2,1);
x2 = P_next(1,1);
y2 = P_next(2,1);

a = (y2 - y1)/-(x2 + x1);
b = 1;
%c = -x1 * (y2 - y1) + y1 * (x2 - x1);


if speed_act ~= 0
    %e = c+b*y1/sqrt((a^2)+(b^2));
    e = error;
    
    cross_track_steering = atan(k * e / speed_act);
    heading_err = atan(-a / b) - yaw;
    %heading_err = 1/(tan(-a/b))-yaw;
    steering = heading_err + cross_track_steering;
end
end

== matlab function Generic_13/CreateBus VhclCtrl/path_planner_MATLAB/MATLAB Function2 ==
  data: Pos_X input; Path_Out output; Pos_Y input; Yaw_Angle input; Path_In input
function Path_Out = Abs2RelNew(Pos_X, Pos_Y, Yaw_Angle, Path_In)
%Rotation matrix from absolute to relativ coordination system
R = [cos(Yaw_Angle) sin(Yaw_Angle); -sin(Yaw_Angle) cos(Yaw_Angle)];

Path_X=Path_In(1,:)-Pos_X;      % Shift the points in to the car position
Path_Y=Path_In(2,:)-Pos_Y;      % Shift the points in to the car position
Path=[Path_X;Path_Y];           % Car Point
Path_Out = R*Path;              % Rotate the shifted Points

== matlab function Generic_13/CreateBus VhclCtrl/path_planner_MATLAB/Path_Calculation_V02 ==
  data: x_car input; closest_point output; y_car input; path_x input; instantaneous_path output; y_path input
function [closest_point, instantaneous_path] = calculate_path(x_car, y_car, path_x, y_path)
% x_car: x position of the car
% y_car: y position of the car
% path: [2x400] matrix representing the path
path = [path_x;y_path];
%Smoothing the Path
x = path(1,:);
y = path(2,:);
% Define the number of points you want to add for interpolation
num_extra_points = 0; % Adjust this value as per your requirements
% Compute the total number of points after interpolation
total_points = numel(x) + num_extra_points;
existing_indices = 1:numel(x);
% Create an array of indices for the interpolated points
interpolated_indices = linspace(1, numel(x), total_points);
% Perform spline interpolation on both x and y coordinates
x_interpolated = spline(existing_indices, x, interpolated_indices);
y_interpolated = spline(existing_indices, y, interpolated_indices);

smoothed_path =vertcat(x_interpolated, y_interpolated);
% smoothed_path = smoothed_path_t';


% Calculate the distance between the car and each point on the path
distances = sqrt((smoothed_path(1,:) - x_car).^2 + (smoothed_path(2,:) - y_car).^2);

% Find the index of the closest point on the path
[~, closest_index] = min(distances);

% Get the closest point on the path
closest_point = smoothed_path(:, closest_index);

% Calculate the distance from the closest point to the beginning of the path
distance_to_start = sqrt(sum((smoothed_path(:,closest_index) - smoothed_path(:,1)).^2));

% Calculate the distance from the closest point to the end of the path
distance_to_end = sqrt(sum((smoothed_path(:,closest_index) - smoothed_path(:,end)).^2));

% Determine the number of points to include in the instantaneous path
num_points = min(size(smoothed_path, 2), 20);

% Initialize the instantaneous_path variable using coder.nullcopy
instantaneous_path = coder.nullcopy(zeros(2, num_points));

if distance_to_start < distance_to_end
    % If the closest point is closer to the beginning of the path than the
    % end, include the points starting from the closest point towards the
    % end of the path
    start_index = closest_index;
    end_index = min(size(smoothed_path, 2), closest_index+num_points-1);
else
    % If the closest point is closer to the end of the path than the
    % beginning, include the points starting from the closest point towards
    % the beginning of the path
    start_index = max(1, closest_index-num_points+1);
    end_index = closest_index;
end

%own 
start_index = closest_index;
if start_index > 11139
    end_index = 11159;
    if start_index > 11149
        start_index = 0;
        end_index=20;
    end
else
    end_index = min(size(smoothed_path, 2), closest_index+num_points-1);
end
%own

temp_path = smoothed_path(:, start_index:end_index);
instantaneous_path(:, num_points-size(temp_path, 2)+1:num_points) = temp_path;

end

== matlab function Generic_13/CreateBus VhclCtrl/A*algoithm/MATLAB Function1 ==
  data: start input; deviation output; target input; obstacles input; pathX output; pathY output
function [deviation, pathX, pathY] = generatePathWithObstacles(start, target, obstacles)
    % A* Path Planning
    function path = astar(start, goal, obstacles)
    % A* algorithm implementation
    
    function path = reconstructPath(parent, current)
    % Reconstruct the path from the parent array
    path_old = current;
    while any(parent(:, 1) == path_old(1) & parent(:, 2) == path_old(2))
        idx = find(parent(:, 1) == path_old(1) & parent(:, 2) == path_old(2), 1);
        path = [parent(idx, :); path_old];
    end
    path = path_old;
end
    function neighbors = generateNeighbors(current, obstacles)
    % Generate neighboring nodes (adjacent and diagonal)
    possibleMoves = [-1, 0; 1, 0; 0, -1; 0, 1; -1, -1; -1, 1; 1, -1; 1, 1];
    neighbors = bsxfun(@plus, current, possibleMoves);

    % Filter out neighbors outside the map
    inMap = neighbors(:, 1) >= 1 & neighbors(:, 1) <= 100 & neighbors(:, 2) >= 1 & neighbors(:, 2) <= 100;
    neighbors = neighbors(inMap, :);
    end
    function result = inSet(position, set)
    % Check if a position is in the set
    result = any(isequal(set(:, 1:2), position), 2);
end

    function result = inObstacles(position, obstacles)
    % Check if a position is in the obstacles
    result = any(isequal(obstacles, position), 2);
    end
    % Parameters
    mapSize = 100; % Adjust as needed
    openSet = zeros(mapSize, 3); % [x, y, f]
    closedSet = zeros(mapSize, 3); % [x, y, f]
    parent = zeros(mapSize, 2); % [parentX, parentY]

    % Functions to calculate heuristic and cost
    heuristic = @(pos, goal) sqrt((pos(1) - goal(1))^2 + (pos(2) - goal(2))^2);
    cost = @(pos, parent) sqrt((pos(1) - parent(1))^2 + (pos(2) - parent(2))^2);

    % Initialize starting point
    openSet(1, :) = [start, heuristic(start, goal)];
    closedSet = zeros(mapSize, 3);

    while any(openSet(:, 1))
        % Find the node with the lowest f in the open set
        [~, currentIdx] = min(openSet(:, 3));
        current = openSet(currentIdx, 1:2);

        % Goal reached
        if isequal(current, goal)
            path = reconstructPath(parent, current);
            return;
        end

        % Move current from openSet to closedSet
        openSet(currentIdx, :) = [0, 0, 0];
        closedSet(currentIdx, :) = [current, heuristic(current, goal)];

        % Generate neighbors
        neighbors = generateNeighbors(current, obstacles);

        for i = 1:size(neighbors, 1)
            neighbor = neighbors(i, :);

            % Skip if in closedSet or obstacle
            if ~inSet(neighbor, closedSet) && ~inObstacles(neighbor, obstacles)
                % Calculate tentative g score
                tentativeG = cost(neighbor, current) + cost(current, start);

                % Check if neighbor is not in openSet or has a better g score
                idxInOpenSet = find(isequal(openSet(:, 1:2), neighbor), 1);
                if isempty(idxInOpenSet) || tentativeG < cost(neighbor, start)
                    % Update parent and g score
                    parent(idxInOpenSet, :) = current;
                    openSet(idxInOpenSet, :) = [neighbor, tentativeG + heuristic(neighbor, goal)];
                end
            end
        end
    end

    % No path found
    path = [];
end
    path = astar(start, target, obstacles);

    % Extract X and Y coordinates from the path
    pathX1 = path(:, 1);
    pathX = pathX1(1);
    pathY1 = path(:, 2);
    pathY = pathY1(1);

    % Calculate deviation from the vehicle to the generated path
    deviation_1 = sqrt((start(1) - pathX).^2 + (start(2) - pathY).^2);
    deviation =deviation_1(1); 
end

== matlab function Generic_13/CreateBus VhclCtrl/Subsystem/MATLAB Function1 ==
  data: x input; path output; y input
function path = fcn(x , y)
path = [x;y];
end

== matlab function Generic_13/CreateBus VhclCtrl/Subsystem1/MATLAB Function ==
  data: vehicleX input; deviationAngle output; vehicleY input; pathX input; pathY input; vehicleYaw input
function deviationAngle = calculateDeviationAngle(vehicleX, vehicleY, pathX, pathY, vehicleYaw)
    % Calculate the vector from the vehicle to the path point
    vectorToPath = [pathX - vehicleX, pathY - vehicleY];

    % Calculate the angle between the vehicle's heading and the vector to the path point
    angleToPath = atan2(vectorToPath(2), vectorToPath(1));

    % Calculate the deviation angle
    deviationAngle = vehicleYaw - angleToPath;

    % Ensure the result is within the range [-pi, pi]
    deviationAngle = mod(deviationAngle + pi, 2*pi) - pi;
end

== matlab function Generic_13/CreateBus VhclCtrl/Stanley  steering & speed//Brake controller/Road sensor set & path planning/Road sensor set & path planning/Car_yaw_rate/calculate_path_curvature2 ==
  data: path_x input; path_curvature output; path_y input
function path_curvature = calculate_path_curvature(path_x, path_y)
    x = path_x;
    y = path_y;
    
    % First and second derivatives
    dx = gradient(x);
    dy = gradient(y);
    
    ddx = gradient(dx);
    ddy = gradient(dy);
    
    % Path curvature with a small constant added to the denominator
    epsilon = 1e-6; % small constant to avoid division by zero
    curvature_denominator = (dx.^2 + dy.^2).^(3/2) + epsilon;
    path_curvature = max((dx .* ddy - dy .* ddx) ./ curvature_denominator);
    
    % Smooth the curvature using a moving average
    window_size = 5; % adjust the window size as needed
    path_curvature = smoothdata(path_curvature, 'movmean', window_size);
end

== matlab function Generic_13/CreateBus VhclCtrl/Stanley  steering & speed//Brake controller/Path_reshaping ==
  data: x input; path_out output; y input
function path_out = full_path(x,y)
path_out= [x;y];

== matlab function Generic_13/CreateBus VhclCtrl/Stanley  steering & speed//Brake controller/Road sensor set & path planning/Road sensor set & path planning/Path_curvature/calculate_path_curvature1 ==
  data: path_x input; path_curvature output; path_y input
function path_curvature = calculate_path_curvature(path_x, path_y)
    x = path_x;
    y = path_y;
    
    % First and second derivatives
    dx = gradient(x);
    dy = gradient(y);
    
    ddx = gradient(dx);
    ddy = gradient(dy);
    
    % Path curvature with a small constant added to the denominator
    epsilon = 1e-6; % small constant to avoid division by zero
    curvature_denominator = (dx.^2 + dy.^2).^(3/2) + epsilon;
    path_curvature = max((dx .* ddy - dy .* ddx) ./ curvature_denominator);
    
    % Smooth the curvature using a moving average
    window_size = 5; % adjust the window size as needed
    path_curvature = smoothdata(path_curvature, 'movmean', window_size);
end
